simulink model "sldemo_counters"  (Simulink 7.6)
settings: Solver=FixedStepDiscrete  StartTime=0.0  StopTime=2.25  FixedStep=.01  RelTol=1e-3  AbsTol=1e-6
Description:
  | Counters Using Conditionally Executed Subsystems
  | 
  | This demonstration uses counter circuits to contrast the execution of blocks in enabled
  | subsystems and triggered subsystems for the same control signal. After running the
  | simulation, the scope shows three plots.
  | 
  | The first of these plots shows the control signal which is the output of the discrete
  | pulse generator.
  | 
  | The second plot shows the output of the counter circuit in the enabled subsystem.
  | The counter increments while the subsystem is enabled and then holds its output when
  | the subsystem is disabled. The counter resets to zero when the subsystem is re-enabled
  | because the enable port was configured to reset states when enabling.
  | 
  | The third plot shows the output of the counter circuit in the triggered subsystem. The
  | counter increments every rising edge of the control signal.
  | 
  | The signals are shown in a Signal Viewer scope that does not require a scope block to
  | be put into the block diagram.  Instead, the "glasses" icon notation on the ports show
  | that a Signal Viewer is attached.  Double click on the glasses to make the Signal
  | Viewer appear if it is hidden.
settings Model: Creator=The MathWorks Inc.  ExtModeTrigMode=oneshot  ExtModeArmWhenConnect=off  ExtModeAutoUpdateStatusClock=off
settings DataIOCC: LimitDataPoints=off
settings OptimizationCC: BlockReduction=off  BooleanDataType=off  InlineInvariantSignals=on  InitFltsAndDblsToZero=on  BufferReusableBoundary=off
settings DebuggingCC: SaveWithParameterizedLinksMsg=none  SignalResolutionControl=TryResolveAllWithWarning  SolverPrmCheckMsg=none  MultiTaskDSMMsg=warning  MultiTaskCondExecSysMsg=none  BusObjectLabelMismatch=none
settings HardwareCC: TargetUnknown=on
settings RTWCC: IncludeERTFirstTime=on
settings GRTTargetCC: TargetFcnLib=ansi_tfl_tmw.mat

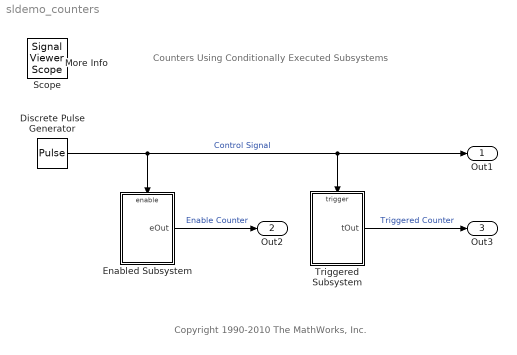
== system sldemo_counters ==
  note: Counters Using
      | Conditionally Executed Subsystems
  note: Copyright 1990-2010 The MathWorks, Inc.
  Discrete Pulse Generator : DiscretePulseGenerator  Period=40  PulseWidth=20  SampleTime=0.01
  Enabled Subsystem : Subsystem  TreatAsAtomicUnit=on
  More Info : Subsystem
      settings: OpenFcn=showdemo(bdroot(gcs))
      mask Display: disp('?')
  Triggered Subsystem : Subsystem  TreatAsAtomicUnit=on
  Out1 : Outport
  Out2 : Outport  Port=2
  Out3 : Outport  Port=3
  Scope : SignalViewerScope  IOType=viewer  NumInputPorts=3  RefreshTime=0.035000
      settings: TimeRange=2.25  YMin=-0.1~0~-0.5  YMax=1.1~20~4.5
  wires:
  Discrete Pulse Generator/1 -> Enabled Subsystem/Enable, Triggered Subsystem/Trigger, Out1/1  "Control Signal"
  Triggered Subsystem/1(tOut) -> Out3/1  "Triggered Counter"
  Enabled Subsystem/1(eOut) -> Out2/1  "Enable Counter"

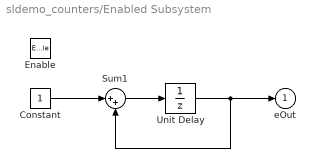
== system sldemo_counters/Enabled Subsystem ==
  Enable : EnablePort  StatesWhenEnabling=reset
  Constant : Constant
  Sum1 : Sum  Inputs=|++  SaturateOnIntegerOverflow=on  InputSameDT=on  OutDataTypeStr=Inherit: Same as first input
  Unit Delay : UnitDelay  SampleTime=.01
  eOut : Outport  InitialOutput=0
  wires:
  Sum1/1 -> Unit Delay/1
  Constant/1 -> Sum1/1
  Unit Delay/1 -> eOut/1, Sum1/2

== system sldemo_counters/More Info ==

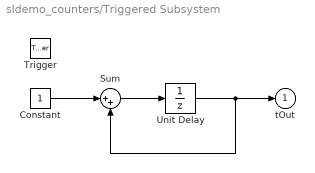
== system sldemo_counters/Triggered Subsystem ==
  Trigger : TriggerPort
  Constant : Constant
  Sum : Sum  Inputs=|++  SaturateOnIntegerOverflow=on  InputSameDT=on  OutDataTypeStr=Inherit: Same as first input
  Unit Delay : UnitDelay  SampleTime=-1
  tOut : Outport  InitialOutput=0
  wires:
  Sum/1 -> Unit Delay/1
  Constant/1 -> Sum/1
  Unit Delay/1 -> tOut/1, Sum/2
